simulink model "Drive_Path_Planning"  (R2020a)
settings: Solver=FixedStepAuto  StartTime=0.0  StopTime=30  FixedStep=0.001  RelTol=1e-3  EnableMultiTasking=on
undefined symbols (not defined in the file): gain, sigbuilder_block, X, x_constant, Y, Z
libraries: sm_lib x168, nesl_utility x16, simulink x8, Contact_Forces_Lib x5
(part 4 of 4)

== system Drive_Path_Planning/Try_Spot_3  ==
  DIAGONAL 2 Return : Subsystem
  Diagonal 2 : Subsystem
  Rectangular Joint3 : sm_lib/Joints/Rectangular Joint  JointMode=Normal  SenseConstraintForce=off  SenseConstraintForceX=off  SenseConstraintForceY=off  SenseConstraintForceZ=off  SenseConstraintTorque=off  SenseConstraintTorqueX=off  SenseConstraintTorqueY=off  SenseConstraintTorqueZ=off  SenseTotalForce=off  SenseTotalForceX=off  SenseTotalForceY=off  SenseTotalForceZ=off  SenseTotalTorque=off  SenseTotalTorqueX=off  SenseTotalTorqueY=off  SenseTotalTorqueZ=off  CompositeWrenchDir=FollowerOnBase  CompositeWrenchFrame=BaseFrame  PxEquilibriumPosition=0  PxEquilibriumPositionUnits=m  PxSpringStiffness=0  PxSpringStiffnessUnits=N/m  PxDampingCoefficient=0  PxDampingCoefficientUnits=N/(m/s)  PxTorqueActuationMode=InputTorque  PxMotionActuationMode=ComputedMotion  PxSensePosition=off  PxSenseVelocity=off  PxSenseAcceleration=off  PxSenseTorqueForce=off  PxSenseLowerLimitTorqueForce=off  PxSenseUpperLimitTorqueForce=off  PxLowerLimitSpecify=off  PxLowerLimitBound=-1  PxLowerLimitBoundUnits=m  PxLowerLimitStiffness=1e6  PxLowerLimitStiffnessUnits=N/m  PxLowerLimitDamping=1e3  PxLowerLimitDampingUnits=N/(m/s)  PxLowerLimitTransitionRegionWidth=1e-4  PxLowerLimitTransitionRegionWidthUnits=m  PxUpperLimitSpecify=off  PxUpperLimitBound=1  PxUpperLimitBoundUnits=m  PxUpperLimitStiffness=1e6  PxUpperLimitStiffnessUnits=N/m  PxUpperLimitDamping=1e3  PxUpperLimitDampingUnits=N/(m/s)  PxUpperLimitTransitionRegionWidth=1e-4  PxUpperLimitTransitionRegionWidthUnits=m  PxPositionTargetSpecify=off  PxPositionTargetPriority=High  PxPositionTargetValue=0  PxPositionTargetValueUnits=m  PxVelocityTargetSpecify=off  PxVelocityTargetPriority=High  PxVelocityTargetValue=0  PxVelocityTargetValueUnits=m/s  PyEquilibriumPosition=0  PyEquilibriumPositionUnits=m  PySpringStiffness=0  PySpringStiffnessUnits=N/m  PyDampingCoefficient=0  PyDampingCoefficientUnits=N/(m/s)  PyTorqueActuationMode=InputTorque  PyMotionActuationMode=ComputedMotion  PySensePosition=off  PySenseVelocity=off  PySenseAcceleration=off  PySenseTorqueForce=off  PySenseLowerLimitTorqueForce=off  PySenseUpperLimitTorqueForce=off  PyLowerLimitSpecify=off  PyLowerLimitBound=-1  PyLowerLimitBoundUnits=m  PyLowerLimitStiffness=1e6  PyLowerLimitStiffnessUnits=N/m  PyLowerLimitDamping=1e3  PyLowerLimitDampingUnits=N/(m/s)  PyLowerLimitTransitionRegionWidth=1e-4  PyLowerLimitTransitionRegionWidthUnits=m  PyUpperLimitSpecify=off  PyUpperLimitBound=1  PyUpperLimitBoundUnits=m  PyUpperLimitStiffness=1e6  PyUpperLimitStiffnessUnits=N/m  PyUpperLimitDamping=1e3  PyUpperLimitDampingUnits=N/(m/s)  PyUpperLimitTransitionRegionWidth=1e-4  PyUpperLimitTransitionRegionWidthUnits=m  PyPositionTargetSpecify=off  PyPositionTargetPriority=High  PyPositionTargetValue=0  PyPositionTargetValueUnits=m  PyVelocityTargetSpecify=off  PyVelocityTargetPriority=High  PyVelocityTargetValue=0  PyVelocityTargetValueUnits=m/s
  Rectangular Joint4 : sm_lib/Joints/Rectangular Joint  JointMode=Normal  SenseConstraintForce=off  SenseConstraintForceX=off  SenseConstraintForceY=off  SenseConstraintForceZ=off  SenseConstraintTorque=off  SenseConstraintTorqueX=off  SenseConstraintTorqueY=off  SenseConstraintTorqueZ=off  SenseTotalForce=off  SenseTotalForceX=off  SenseTotalForceY=off  SenseTotalForceZ=off  SenseTotalTorque=off  SenseTotalTorqueX=off  SenseTotalTorqueY=off  SenseTotalTorqueZ=off  CompositeWrenchDir=FollowerOnBase  CompositeWrenchFrame=BaseFrame  PxEquilibriumPosition=0  PxEquilibriumPositionUnits=m  PxSpringStiffness=0  PxSpringStiffnessUnits=N/m  PxDampingCoefficient=0  PxDampingCoefficientUnits=N/(m/s)  PxTorqueActuationMode=InputTorque  PxMotionActuationMode=ComputedMotion  PxSensePosition=off  PxSenseVelocity=off  PxSenseAcceleration=off  PxSenseTorqueForce=off  PxSenseLowerLimitTorqueForce=off  PxSenseUpperLimitTorqueForce=off  PxLowerLimitSpecify=off  PxLowerLimitBound=-1  PxLowerLimitBoundUnits=m  PxLowerLimitStiffness=1e6  PxLowerLimitStiffnessUnits=N/m  PxLowerLimitDamping=1e3  PxLowerLimitDampingUnits=N/(m/s)  PxLowerLimitTransitionRegionWidth=1e-4  PxLowerLimitTransitionRegionWidthUnits=m  PxUpperLimitSpecify=off  PxUpperLimitBound=1  PxUpperLimitBoundUnits=m  PxUpperLimitStiffness=1e6  PxUpperLimitStiffnessUnits=N/m  PxUpperLimitDamping=1e3  PxUpperLimitDampingUnits=N/(m/s)  PxUpperLimitTransitionRegionWidth=1e-4  PxUpperLimitTransitionRegionWidthUnits=m  PxPositionTargetSpecify=off  PxPositionTargetPriority=High  PxPositionTargetValue=0  PxPositionTargetValueUnits=m  PxVelocityTargetSpecify=off  PxVelocityTargetPriority=High  PxVelocityTargetValue=0  PxVelocityTargetValueUnits=m/s  PyEquilibriumPosition=0  PyEquilibriumPositionUnits=m  PySpringStiffness=0  PySpringStiffnessUnits=N/m  PyDampingCoefficient=0  PyDampingCoefficientUnits=N/(m/s)  PyTorqueActuationMode=InputTorque  PyMotionActuationMode=ComputedMotion  PySensePosition=off  PySenseVelocity=off  PySenseAcceleration=off  PySenseTorqueForce=off  PySenseLowerLimitTorqueForce=off  PySenseUpperLimitTorqueForce=off  PyLowerLimitSpecify=off  PyLowerLimitBound=-1  PyLowerLimitBoundUnits=m  PyLowerLimitStiffness=1e6  PyLowerLimitStiffnessUnits=N/m  PyLowerLimitDamping=1e3  PyLowerLimitDampingUnits=N/(m/s)  PyLowerLimitTransitionRegionWidth=1e-4  PyLowerLimitTransitionRegionWidthUnits=m  PyUpperLimitSpecify=off  PyUpperLimitBound=1  PyUpperLimitBoundUnits=m  PyUpperLimitStiffness=1e6  PyUpperLimitStiffnessUnits=N/m  PyUpperLimitDamping=1e3  PyUpperLimitDampingUnits=N/(m/s)  PyUpperLimitTransitionRegionWidth=1e-4  PyUpperLimitTransitionRegionWidthUnits=m  PyPositionTargetSpecify=off  PyPositionTargetPriority=High  PyPositionTargetValue=0  PyPositionTargetValueUnits=m  PyVelocityTargetSpecify=off  PyVelocityTargetPriority=High  PyVelocityTargetValue=0  PyVelocityTargetValueUnits=m/s
  Simulink-PS Converter{5..8} (4 alike) : nesl_utility/Simulink-PS Converter  PhysicalDomain=network_engine_domain  SubClassName=ps_input  LeftPortType=input  RightPortType=output  PseudoPeriodic=off  Frequencies=[]  NoiseDistribution=none  NoiseParameters=[]  Unit=1  AffineConversion=off  FilteringAndDerivatives=provide  SimscapeFilterOrder=1  InputFilterTimeConstant=0.001  UdotUserProvided=0
  Terminator2 : Terminator
  Terminator3 : Terminator
  Conn1 : PMIOPort  Side=Left
  Conn2 : PMIOPort  Port=2  Side=Right
  Conn3 : PMIOPort  Port=3  Side=Left
  Conn4 : PMIOPort  Port=4  Side=Right
  wires:
  Diagonal 2/3(Out3) -> Simulink-PS Converter5/1
  DIAGONAL 2 Return/3(Out3) -> Simulink-PS Converter7/1
  Diagonal 2/4(Out4) -> Simulink-PS Converter6/1
  Diagonal 2/2(Out2) -> Terminator2/1
  Diagonal 2/1(Out1) -> Terminator3/1
  DIAGONAL 2 Return/4(Out4) -> Simulink-PS Converter8/1
  connections:
  Rectangular Joint3/RConn1 -- Conn2/RConn1
  Simulink-PS Converter6/RConn1 -- Rectangular Joint3/LConn3
  Simulink-PS Converter8/RConn1 -- Rectangular Joint4/LConn3
  Rectangular Joint4/LConn1 -- Conn3/RConn1
  Simulink-PS Converter5/RConn1 -- Rectangular Joint3/LConn2
  Simulink-PS Converter7/RConn1 -- Rectangular Joint4/LConn2
  Rectangular Joint4/RConn1 -- Conn4/RConn1
  Rectangular Joint3/LConn1 -- Conn1/RConn1

== system Drive_Path_Planning/Try_Spot_4 ==
  EQUATION PAth1 : Subsystem
  Equation Curve CONSTANT1 : Subsystem
  Rectangular Joint7 : sm_lib/Joints/Rectangular Joint  JointMode=Normal  SenseConstraintForce=off  SenseConstraintForceX=off  SenseConstraintForceY=off  SenseConstraintForceZ=off  SenseConstraintTorque=off  SenseConstraintTorqueX=off  SenseConstraintTorqueY=off  SenseConstraintTorqueZ=off  SenseTotalForce=off  SenseTotalForceX=off  SenseTotalForceY=off  SenseTotalForceZ=off  SenseTotalTorque=off  SenseTotalTorqueX=off  SenseTotalTorqueY=off  SenseTotalTorqueZ=off  CompositeWrenchDir=FollowerOnBase  CompositeWrenchFrame=BaseFrame  PxEquilibriumPosition=0  PxEquilibriumPositionUnits=m  PxSpringStiffness=0  PxSpringStiffnessUnits=N/m  PxDampingCoefficient=0  PxDampingCoefficientUnits=N/(m/s)  PxTorqueActuationMode=InputTorque  PxMotionActuationMode=ComputedMotion  PxSensePosition=off  PxSenseVelocity=off  PxSenseAcceleration=off  PxSenseTorqueForce=off  PxSenseLowerLimitTorqueForce=off  PxSenseUpperLimitTorqueForce=off  PxLowerLimitSpecify=off  PxLowerLimitBound=-1  PxLowerLimitBoundUnits=m  PxLowerLimitStiffness=1e6  PxLowerLimitStiffnessUnits=N/m  PxLowerLimitDamping=1e3  PxLowerLimitDampingUnits=N/(m/s)  PxLowerLimitTransitionRegionWidth=1e-4  PxLowerLimitTransitionRegionWidthUnits=m  PxUpperLimitSpecify=off  PxUpperLimitBound=6.1  PxUpperLimitBoundUnits=m  PxUpperLimitStiffness=1e10  PxUpperLimitStiffnessUnits=N/m  PxUpperLimitDamping=1e3  PxUpperLimitDampingUnits=N/(m/s)  PxUpperLimitTransitionRegionWidth=1e-4  PxUpperLimitTransitionRegionWidthUnits=m  PxPositionTargetSpecify=off  PxPositionTargetPriority=High  PxPositionTargetValue=0  PxPositionTargetValueUnits=m  PxVelocityTargetSpecify=off  PxVelocityTargetPriority=High  PxVelocityTargetValue=0  PxVelocityTargetValueUnits=m/s  PyEquilibriumPosition=0  PyEquilibriumPositionUnits=m  PySpringStiffness=0  PySpringStiffnessUnits=N/m  PyDampingCoefficient=0  PyDampingCoefficientUnits=N/(m/s)  PyTorqueActuationMode=InputTorque  PyMotionActuationMode=ComputedMotion  PySensePosition=off  PySenseVelocity=off  PySenseAcceleration=off  PySenseTorqueForce=off  PySenseLowerLimitTorqueForce=off  PySenseUpperLimitTorqueForce=off  PyLowerLimitSpecify=off  PyLowerLimitBound=-1  PyLowerLimitBoundUnits=m  PyLowerLimitStiffness=1e6  PyLowerLimitStiffnessUnits=N/m  PyLowerLimitDamping=1e3  PyLowerLimitDampingUnits=N/(m/s)  PyLowerLimitTransitionRegionWidth=1e-4  PyLowerLimitTransitionRegionWidthUnits=m  PyUpperLimitSpecify=off  PyUpperLimitBound=8.455  PyUpperLimitBoundUnits=m  PyUpperLimitStiffness=1e6  PyUpperLimitStiffnessUnits=N/m  PyUpperLimitDamping=1e3  PyUpperLimitDampingUnits=N/(m/s)  PyUpperLimitTransitionRegionWidth=1e-4  PyUpperLimitTransitionRegionWidthUnits=m  PyPositionTargetSpecify=off  PyPositionTargetPriority=High  PyPositionTargetValue=0  PyPositionTargetValueUnits=m  PyVelocityTargetSpecify=off  PyVelocityTargetPriority=High  PyVelocityTargetValue=1.1  PyVelocityTargetValueUnits=m/s
  Simulink-PS Converter10 : nesl_utility/Simulink-PS Converter  PhysicalDomain=network_engine_domain  SubClassName=ps_input  LeftPortType=input  RightPortType=output  PseudoPeriodic=off  Frequencies=[]  NoiseDistribution=none  NoiseParameters=[]  Unit=1  AffineConversion=off  FilteringAndDerivatives=provide  SimscapeFilterOrder=1  InputFilterTimeConstant=0.001  UdotUserProvided=0
  Conn1 : PMIOPort  Side=Right
  Conn2 : PMIOPort  Port=2  Side=Left
  Conn3 : PMIOPort  Port=3  Side=Left
  wires:
  EQUATION PAth1/1(Out1) -> Simulink-PS Converter10/1
  connections:
  Simulink-PS Converter10/RConn1 -- Rectangular Joint7/LConn3
  Rectangular Joint7/LConn1 -- Conn2/RConn1
  Equation Curve CONSTANT1/RConn1 -- Rectangular Joint7/LConn2
  Rectangular Joint7/RConn1 -- Conn1/RConn1
  EQUATION PAth1/LConn1 -- Conn3/RConn1

== system Drive_Path_Planning/ /Signal Builder ==
  Demux : Demux  Tag=STV Demux  Outputs=2
      settings: DisplayOption=none
  FromWs : FromWorkspace  Tag=STV FromWs  VariableName=tuvar
      SigBuilderData=|
      | common.afterFinalStr = 'Extrapolate'
      | common.sampleTime = 0
      | dataSet.timeRange = [0 10]
      | dataSet.name = 'Group 1'
      | sbobj.Groups.Name = 'Group 1'
      | sbobj.Groups.Signals(1).Name = 'S2'
      | sbobj.Groups.Signals(1).XData = [0 0.4 0.4 5 5 10]
      | sbobj.Groups.Signals(1).YData = [0 0 -0.02 -0.02 0 0]
      | sbobj.Groups.Signals(2).Name = '1'
      | sbobj.Groups.Signals(2).XData = [0 0.2 0.2 0.4 0.4 10]
      | sbobj.Groups.Signals(2).YData = [0 0 10 10 0 0]
  S2 : Outport  Tag=STV Outport
  1 : Outport  Tag=STV Outport  Port=2
  wires:
  FromWs/1 -> Demux/1
  Demux/1 -> S2/1
  Demux/2 -> 1/1

== system Drive_Path_Planning/ Try_Spot_5 /EQUATION PAth ==
  Clock4 : Clock
  If Action Subsystem6 : Subsystem  TreatAsAtomicUnit=on
  If5 : If  IfExpression=u1>20
  Multiply1 : Gain  Gain=gain
  Subsystem5 : Subsystem
  Subsystem6 : Subsystem
  Subsystem7 : Subsystem
  Conn1 : PMIOPort  Side=Left
  Out1 : Outport
  Out2 : Outport  Port=2
  wires:
  Multiply1/1 -> If Action Subsystem6/1(In1)
  Subsystem5/1(Out1) -> Subsystem6/1(In1)
  If5/1 -> If Action Subsystem6/Action
  Subsystem6/1(Out1) -> Subsystem7/1(In1)
  Subsystem7/1(Out1) -> Multiply1/1
  If5/2 -> Out2/1
  Clock4/1 -> If5/1
  If Action Subsystem6/1(Out1) -> Out1/1
  connections:
  Subsystem5/LConn1 -- Conn1/RConn1

== system Drive_Path_Planning/ Try_Spot_5 /Equation Curve CONSTANT ==
  Clock1 : Clock
  Constant7 : Constant  Value=38
  If Action Subsystem3 : Subsystem  TreatAsAtomicUnit=on
  If3 : If  IfExpression=u1 > 20
  Product4 : Product
  Signal Builder4 : Subsystem  Tag=STV Subsys  LoadFcn=sigbuilder_block('load');  StartFcn=sigbuilder_block('start');  StopFcn=sigbuilder_block('stop');  ClipboardFcn=sigbuilder_block('clipboard');  mask(Sigbuilder block){tuvar=[0:10]}
      mask help: Simulink:masks:SigbuilderBlock_MD
      mask init:
      | if ~strcmp(get_param(bdroot(gcbh),'SimulationStatus'),'stopped') tuvar = sigbuilder_block('maskInit'); end
      settings: CopyFcn=sigbuilder_block('copy');  DeleteFcn=sigbuilder_block('delete');  ModelCloseFcn=sigbuilder_block('modelClose');  PreSaveFcn=sigbuilder_block('preSave');  PauseFcn=sigbuilder_block('pause');  ContinueFcn=sigbuilder_block('continue');  NameChangeFcn=sigbuilder_block('namechange');  OpenFcn=sigbuilder_block('open',[437.6 153 550.4 359.25 ]);  CloseFcn=sigbuilder_block('close');
      mask Display: plot(0, 0, 100, 100,[2, 2, 32, 32, 2], [68, 8, 8, 68, 68],[32, 2], [38, 38], [32, 19, 2],[53, 60, 44], [32, 17, 17, 2],[16, 16, 31, 31]);txt = getActiveGroup(gcbh);text(2, 100, txt,'verticalAlignment', 'top');
  Simulink-PS Converter11 : nesl_utility/Simulink-PS Converter  PhysicalDomain=network_engine_domain  SubClassName=ps_input  LeftPortType=input  RightPortType=output  PseudoPeriodic=off  Frequencies=[]  NoiseDistribution=none  NoiseParameters=[]  Unit=1  AffineConversion=off  FilteringAndDerivatives=provide  SimscapeFilterOrder=1  InputFilterTimeConstant=0.001  UdotUserProvided=0
  Conn1 : PMIOPort  Side=Right
  Out1 : Outport
  wires:
  Product4/1 -> If Action Subsystem3/1(In1)
  If3/1 -> If Action Subsystem3/Action
  Constant7/1 -> Product4/2
  Clock1/1 -> If3/1
  Signal Builder4/1(Signal 1) -> Product4/1
  If3/2 -> Out1/1
  If Action Subsystem3/1(Out1) -> Simulink-PS Converter11/1
  connections:
  Simulink-PS Converter11/RConn1 -- Conn1/RConn1

== system Drive_Path_Planning/BOT/Friction_Wheel_1 ==
  Sphere to Plane Force : Contact_Forces_Lib/3D/Sphere to Plane Force  sphere_rad=0.063  plane_lenx=13.3  plane_leny=10  plane_depth=0.00005  force_law=Linear  k_contact=1e4  b_contact=1e2  pen_full_damp_F=1e-4  pen_exponent=1  custom_param_1=1  custom_param_2=1  friction_law=Stick-Slip Continuous  mu_kinetic=friction  mu_static=0.4  v_thr=0.1  vis_on=off  vis_opc_en=0  vis_len_plaBz=0.005  vis_clr=[0.9 0.2 0.2]  vis_opc=0.7
  Terminator : Terminator
  Conn2 : PMIOPort  Side=Left
  Cylindrical Solid26 : PMIOPort  Port=2  Side=Left
  wires:
  Sphere to Plane Force/1 -> Terminator/1
  connections:
  Sphere to Plane Force/RConn1 -- Conn2/RConn1
  Cylindrical Solid26/RConn1 -- Sphere to Plane Force/LConn1

== system Drive_Path_Planning/BOT/Friction_Wheel_2 ==
  Sphere to Plane Force1 : Contact_Forces_Lib/3D/Sphere to Plane Force  sphere_rad=0.063  plane_lenx=13.3  plane_leny=10  plane_depth=0.00005  force_law=Linear  k_contact=1e4  b_contact=1e2  pen_full_damp_F=1e-4  pen_exponent=1  custom_param_1=1  custom_param_2=1  friction_law=Stick-Slip Continuous  mu_kinetic=friction  mu_static=0.4  v_thr=0.1  vis_on=off  vis_opc_en=0  vis_len_plaBz=0.005  vis_clr=[0.9 0.2 0.2]  vis_opc=0.7
  Sphere to Plane Force3 : Contact_Forces_Lib/3D/Sphere to Plane Force  sphere_rad=0.78  plane_lenx=0.8005  plane_leny=1.2375  plane_depth=0.05  force_law=Linear  k_contact=1e4  b_contact=1e2  pen_full_damp_F=1e-4  pen_exponent=1  custom_param_1=1  custom_param_2=1  friction_law=Stick-Slip Continuous  mu_kinetic=friction_1  mu_static=0.09  v_thr=0.001  vis_on=off  vis_opc_en=0  vis_len_plaBz=0.005  vis_clr=[0.9 0.2 0.2]  vis_opc=0.7
  Terminator1 : Terminator
  Terminator3 : Terminator
  Conn4 : PMIOPort  Side=Left
  Connection Port : PMIOPort  Port=2  Side=Left
  Cylindrical Solid26 : PMIOPort  Port=3  Side=Left
  wires:
  Sphere to Plane Force1/1 -> Terminator1/1
  Sphere to Plane Force3/1 -> Terminator3/1
  connections:
  Sphere to Plane Force1/LConn1 -- Cylindrical Solid26/RConn1 -- Sphere to Plane Force3/LConn1
  Sphere to Plane Force3/RConn1 -- Connection Port/RConn1
  Conn4/RConn1 -- Sphere to Plane Force1/RConn1

== system Drive_Path_Planning/BOT/Friction_Wheel_3 ==
  Sphere to Plane Force2 : Contact_Forces_Lib/3D/Sphere to Plane Force  sphere_rad=0.063  plane_lenx=13.3  plane_leny=10  plane_depth=0.00005  force_law=Linear  k_contact=1e4  b_contact=1e2  pen_full_damp_F=1e-4  pen_exponent=1  custom_param_1=1  custom_param_2=1  friction_law=Stick-Slip Continuous  mu_kinetic=friction  mu_static=0.4  v_thr=0.1  vis_on=off  vis_opc_en=0  vis_len_plaBz=0.005  vis_clr=[0.9 0.2 0.2]  vis_opc=0.7
  Sphere to Plane Force4 : Contact_Forces_Lib/3D/Sphere to Plane Force  sphere_rad=0.7  plane_lenx=1.2375  plane_leny=1.2375  plane_depth=0.05  force_law=Linear  k_contact=1e4  b_contact=1e2  pen_full_damp_F=1e-4  pen_exponent=1  custom_param_1=1  custom_param_2=1  friction_law=Stick-Slip Continuous  mu_kinetic=friction_2  mu_static=0.09  v_thr=0.001  vis_on=off  vis_opc_en=0  vis_len_plaBz=0.005  vis_clr=[0.9 0.2 0.2]  vis_opc=0.7
  Terminator : Terminator
  Terminator2 : Terminator
  Cylindrical Solid27 : PMIOPort  Side=Left
  Conn3 : PMIOPort  Port=2  Side=Left
  Conn5 : PMIOPort  Port=3  Side=Left
  wires:
  Sphere to Plane Force2/1 -> Terminator2/1
  Sphere to Plane Force4/1 -> Terminator/1
  connections:
  Sphere to Plane Force2/LConn1 -- Cylindrical Solid27/RConn1 -- Sphere to Plane Force4/LConn1
  Conn3/RConn1 -- Sphere to Plane Force2/RConn1
  Conn5/RConn1 -- Sphere to Plane Force4/RConn1

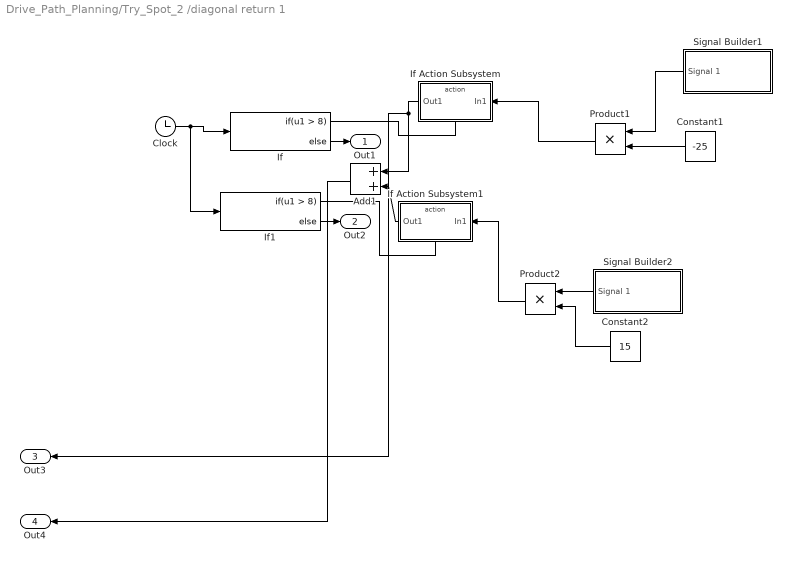
== system Drive_Path_Planning/Try_Spot_2 /diagonal return 1 ==
  Add1 : Sum
  Clock : Clock
  Constant1 : Constant  Value=-25
  Constant2 : Constant  Value=15
  If : If  IfExpression=u1 > 8
  If Action Subsystem : Subsystem  TreatAsAtomicUnit=on
  If Action Subsystem1 : Subsystem  TreatAsAtomicUnit=on
  If1 : If  IfExpression=u1 > 8
  Product1 : Product
  Product2 : Product
  Signal Builder1 : Subsystem  Tag=STV Subsys  LoadFcn=sigbuilder_block('load');  StartFcn=sigbuilder_block('start');  StopFcn=sigbuilder_block('stop');  ClipboardFcn=sigbuilder_block('clipboard');  mask(Sigbuilder block){tuvar=[0:10]}
      mask help: Simulink:masks:SigbuilderBlock_MD
      mask init:
      | if ~strcmp(get_param(bdroot(gcbh),'SimulationStatus'),'stopped') tuvar = sigbuilder_block('maskInit'); end
      settings: CopyFcn=sigbuilder_block('copy');  DeleteFcn=sigbuilder_block('delete');  ModelCloseFcn=sigbuilder_block('modelClose');  PreSaveFcn=sigbuilder_block('preSave');  PauseFcn=sigbuilder_block('pause');  ContinueFcn=sigbuilder_block('continue');  NameChangeFcn=sigbuilder_block('namechange');  OpenFcn=sigbuilder_block('open',[437.6 153 550.4 359.25 ]);  CloseFcn=sigbuilder_block('close');
      mask Display: plot(0, 0, 100, 100,[2, 2, 32, 32, 2], [68, 8, 8, 68, 68],[32, 2], [38, 38], [32, 19, 2],[53, 60, 44], [32, 17, 17, 2],[16, 16, 31, 31]);txt = getActiveGroup(gcbh);text(2, 100, txt,'verticalAlignment', 'top');
  Signal Builder2 : Subsystem  Tag=STV Subsys  LoadFcn=sigbuilder_block('load');  StartFcn=sigbuilder_block('start');  StopFcn=sigbuilder_block('stop');  ClipboardFcn=sigbuilder_block('clipboard');  mask(Sigbuilder block){tuvar=[0:10]}
      mask help: Simulink:masks:SigbuilderBlock_MD
      mask init:
      | if ~strcmp(get_param(bdroot(gcbh),'SimulationStatus'),'stopped') tuvar = sigbuilder_block('maskInit'); end
      settings: CopyFcn=sigbuilder_block('copy');  DeleteFcn=sigbuilder_block('delete');  ModelCloseFcn=sigbuilder_block('modelClose');  PreSaveFcn=sigbuilder_block('preSave');  PauseFcn=sigbuilder_block('pause');  ContinueFcn=sigbuilder_block('continue');  NameChangeFcn=sigbuilder_block('namechange');  OpenFcn=sigbuilder_block('open',[437.6 153 550.4 359.25 ]);  CloseFcn=sigbuilder_block('close');
      mask Display: plot(0, 0, 100, 100,[2, 2, 32, 32, 2], [68, 8, 8, 68, 68],[32, 2], [38, 38], [32, 19, 2],[53, 60, 44], [32, 17, 17, 2],[16, 16, 31, 31]);txt = getActiveGroup(gcbh);text(2, 100, txt,'verticalAlignment', 'top');
  Out1 : Outport
  Out2 : Outport  Port=2
  Out3 : Outport  Port=3
  Out4 : Outport  Port=4
  wires:
  Constant1/1 -> Product1/2
  If Action Subsystem1/1(Out1) -> Add1/2
  Signal Builder2/1(Signal 1) -> Product2/1
  If/2 -> Out1/1
  Product2/1 -> If Action Subsystem1/1(In1)
  If Action Subsystem/1(Out1) -> Out3/1, Add1/1
  Constant2/1 -> Product2/2
  Product1/1 -> If Action Subsystem/1(In1)
  Add1/1 -> Out4/1
  Clock/1 -> If1/1, If/1
  Signal Builder1/1(Signal 1) -> Product1/1
  If1/2 -> Out2/1
  If/1 -> If Action Subsystem/Action
  If1/1 -> If Action Subsystem1/Action

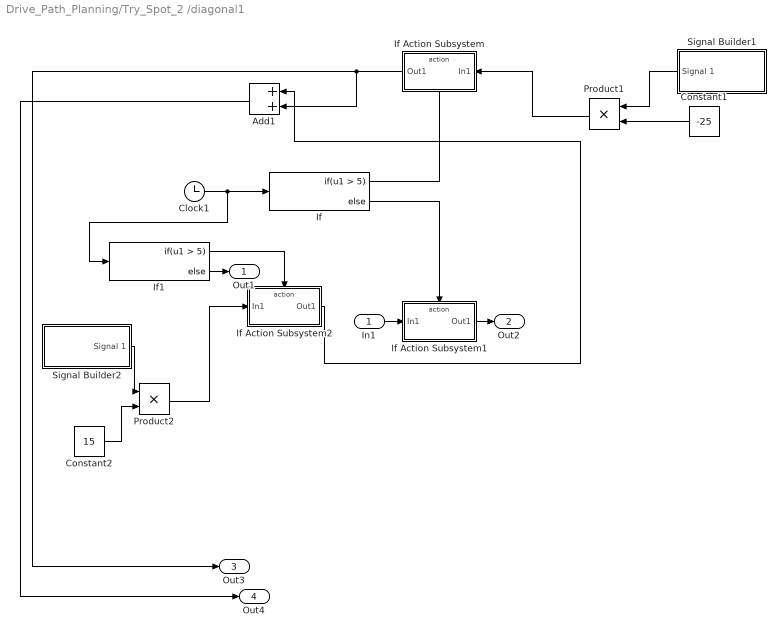
== system Drive_Path_Planning/Try_Spot_2 /diagonal1 ==
  In1 : Inport
  Add1 : Sum
  Clock1 : Clock
  Constant1 : Constant  Value=-25
  Constant2 : Constant  Value=15
  If : If  IfExpression=u1 > 5
  If Action Subsystem : Subsystem  TreatAsAtomicUnit=on
  If Action Subsystem1 : Subsystem  TreatAsAtomicUnit=on
  If Action Subsystem2 : Subsystem  TreatAsAtomicUnit=on
  If1 : If  IfExpression=u1 > 5
  Product1 : Product
  Product2 : Product
  Signal Builder1 : Subsystem  Tag=STV Subsys  LoadFcn=sigbuilder_block('load');  StartFcn=sigbuilder_block('start');  StopFcn=sigbuilder_block('stop');  ClipboardFcn=sigbuilder_block('clipboard');  mask(Sigbuilder block){tuvar=[0:10]}
      mask help: Simulink:masks:SigbuilderBlock_MD
      mask init:
      | if ~strcmp(get_param(bdroot(gcbh),'SimulationStatus'),'stopped') tuvar = sigbuilder_block('maskInit'); end
      settings: CopyFcn=sigbuilder_block('copy');  DeleteFcn=sigbuilder_block('delete');  ModelCloseFcn=sigbuilder_block('modelClose');  PreSaveFcn=sigbuilder_block('preSave');  PauseFcn=sigbuilder_block('pause');  ContinueFcn=sigbuilder_block('continue');  NameChangeFcn=sigbuilder_block('namechange');  OpenFcn=sigbuilder_block('open',[437.6 153 550.4 359.25 ]);  CloseFcn=sigbuilder_block('close');
      mask Display: plot(0, 0, 100, 100,[2, 2, 32, 32, 2], [68, 8, 8, 68, 68],[32, 2], [38, 38], [32, 19, 2],[53, 60, 44], [32, 17, 17, 2],[16, 16, 31, 31]);txt = getActiveGroup(gcbh);text(2, 100, txt,'verticalAlignment', 'top');
  Signal Builder2 : Subsystem  Tag=STV Subsys  LoadFcn=sigbuilder_block('load');  StartFcn=sigbuilder_block('start');  StopFcn=sigbuilder_block('stop');  ClipboardFcn=sigbuilder_block('clipboard');  mask(Sigbuilder block){tuvar=[0:10]}
      mask help: Simulink:masks:SigbuilderBlock_MD
      mask init:
      | if ~strcmp(get_param(bdroot(gcbh),'SimulationStatus'),'stopped') tuvar = sigbuilder_block('maskInit'); end
      settings: CopyFcn=sigbuilder_block('copy');  DeleteFcn=sigbuilder_block('delete');  ModelCloseFcn=sigbuilder_block('modelClose');  PreSaveFcn=sigbuilder_block('preSave');  PauseFcn=sigbuilder_block('pause');  ContinueFcn=sigbuilder_block('continue');  NameChangeFcn=sigbuilder_block('namechange');  OpenFcn=sigbuilder_block('open',[437.6 153 550.4 359.25 ]);  CloseFcn=sigbuilder_block('close');
      mask Display: plot(0, 0, 100, 100,[2, 2, 32, 32, 2], [68, 8, 8, 68, 68],[32, 2], [38, 38], [32, 19, 2],[53, 60, 44], [32, 17, 17, 2],[16, 16, 31, 31]);txt = getActiveGroup(gcbh);text(2, 100, txt,'verticalAlignment', 'top');
  Out1 : Outport
  Out2 : Outport  Port=2
  Out3 : Outport  Port=3
  Out4 : Outport  Port=4
  wires:
  Product2/1 -> If Action Subsystem2/1(In1)
  If Action Subsystem/1(Out1) -> Out3/1, Add1/2
  If/1 -> If Action Subsystem/Action
  Clock1/1 -> If1/1, If/1
  If/2 -> If Action Subsystem1/Action
  Signal Builder2/1(Signal 1) -> Product2/1
  If1/1 -> If Action Subsystem2/Action
  If Action Subsystem2/1(Out1) -> Add1/1
  In1/1 -> If Action Subsystem1/1(In1)
  Constant1/1 -> Product1/2
  Product1/1 -> If Action Subsystem/1(In1)
  Constant2/1 -> Product2/2
  Signal Builder1/1(Signal 1) -> Product1/1
  Add1/1 -> Out4/1
  If Action Subsystem1/1(Out1) -> Out2/1
  If1/2 -> Out1/1

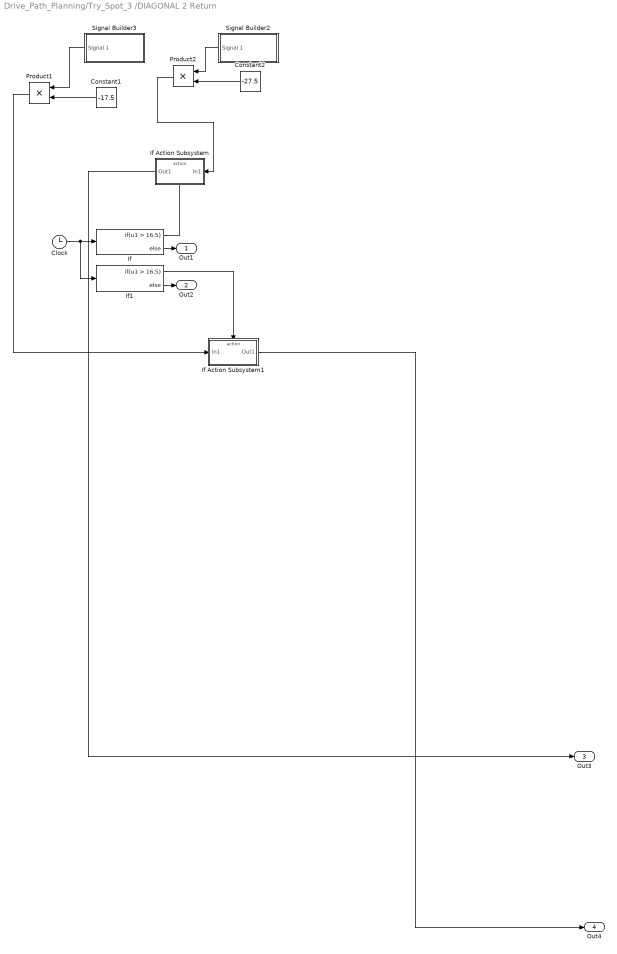
== system Drive_Path_Planning/Try_Spot_3 /DIAGONAL 2 Return ==
  Clock : Clock
  Constant1 : Constant  Value=-17.5
  Constant2 : Constant  Value=-27.5
  If : If  IfExpression=u1 > 16.5
  If Action Subsystem : Subsystem  TreatAsAtomicUnit=on
  If Action Subsystem1 : Subsystem  TreatAsAtomicUnit=on
  If1 : If  IfExpression=u1 > 16.5
  Product1 : Product
  Product2 : Product
  Signal Builder2 : Subsystem  Tag=STV Subsys  LoadFcn=sigbuilder_block('load');  StartFcn=sigbuilder_block('start');  StopFcn=sigbuilder_block('stop');  ClipboardFcn=sigbuilder_block('clipboard');  mask(Sigbuilder block){tuvar=[0:10]}
      mask help: Simulink:masks:SigbuilderBlock_MD
      mask init:
      | if ~strcmp(get_param(bdroot(gcbh),'SimulationStatus'),'stopped') tuvar = sigbuilder_block('maskInit'); end
      settings: CopyFcn=sigbuilder_block('copy');  DeleteFcn=sigbuilder_block('delete');  ModelCloseFcn=sigbuilder_block('modelClose');  PreSaveFcn=sigbuilder_block('preSave');  PauseFcn=sigbuilder_block('pause');  ContinueFcn=sigbuilder_block('continue');  NameChangeFcn=sigbuilder_block('namechange');  OpenFcn=sigbuilder_block('open',[437.6 153 550.4 359.25 ]);  CloseFcn=sigbuilder_block('close');
      mask Display: plot(0, 0, 100, 100,[2, 2, 32, 32, 2], [68, 8, 8, 68, 68],[32, 2], [38, 38], [32, 19, 2],[53, 60, 44], [32, 17, 17, 2],[16, 16, 31, 31]);txt = getActiveGroup(gcbh);text(2, 100, txt,'verticalAlignment', 'top');
  Signal Builder3 : Subsystem  Tag=STV Subsys  LoadFcn=sigbuilder_block('load');  StartFcn=sigbuilder_block('start');  StopFcn=sigbuilder_block('stop');  ClipboardFcn=sigbuilder_block('clipboard');  mask(Sigbuilder block){tuvar=[0:10]}
      mask help: Simulink:masks:SigbuilderBlock_MD
      mask init:
      | if ~strcmp(get_param(bdroot(gcbh),'SimulationStatus'),'stopped') tuvar = sigbuilder_block('maskInit'); end
      settings: CopyFcn=sigbuilder_block('copy');  DeleteFcn=sigbuilder_block('delete');  ModelCloseFcn=sigbuilder_block('modelClose');  PreSaveFcn=sigbuilder_block('preSave');  PauseFcn=sigbuilder_block('pause');  ContinueFcn=sigbuilder_block('continue');  NameChangeFcn=sigbuilder_block('namechange');  OpenFcn=sigbuilder_block('open',[437.6 153 550.4 359.25 ]);  CloseFcn=sigbuilder_block('close');
      mask Display: plot(0, 0, 100, 100,[2, 2, 32, 32, 2], [68, 8, 8, 68, 68],[32, 2], [38, 38], [32, 19, 2],[53, 60, 44], [32, 17, 17, 2],[16, 16, 31, 31]);txt = getActiveGroup(gcbh);text(2, 100, txt,'verticalAlignment', 'top');
  Out1 : Outport
  Out2 : Outport  Port=2
  Out3 : Outport  Port=3
  Out4 : Outport  Port=4
  wires:
  Signal Builder3/1(Signal 1) -> Product1/1
  Constant1/1 -> Product1/2
  If1/1 -> If Action Subsystem1/Action
  Product1/1 -> If Action Subsystem1/1(In1)
  If/1 -> If Action Subsystem/Action
  Clock/1 -> If1/1, If/1
  Product2/1 -> If Action Subsystem/1(In1)
  If/2 -> Out1/1
  Constant2/1 -> Product2/2
  Signal Builder2/1(Signal 1) -> Product2/1
  If1/2 -> Out2/1
  If Action Subsystem1/1(Out1) -> Out4/1
  If Action Subsystem/1(Out1) -> Out3/1

== system Drive_Path_Planning/Try_Spot_3 /Diagonal 2 ==
  Clock : Clock
  Constant1 : Constant  Value=-17
  Constant2 : Constant  Value=-25
  If : If  IfExpression=u1 > 13
  If Action Subsystem : Subsystem  TreatAsAtomicUnit=on
  If Action Subsystem1 : Subsystem  TreatAsAtomicUnit=on
  If1 : If  IfExpression=u1 > 13
  Product1 : Product
  Product2 : Product
  Signal Builder1 : Subsystem  Tag=STV Subsys  LoadFcn=sigbuilder_block('load');  StartFcn=sigbuilder_block('start');  StopFcn=sigbuilder_block('stop');  ClipboardFcn=sigbuilder_block('clipboard');  mask(Sigbuilder block){tuvar=[0:10]}
      mask help: Simulink:masks:SigbuilderBlock_MD
      mask init:
      | if ~strcmp(get_param(bdroot(gcbh),'SimulationStatus'),'stopped') tuvar = sigbuilder_block('maskInit'); end
      settings: CopyFcn=sigbuilder_block('copy');  DeleteFcn=sigbuilder_block('delete');  ModelCloseFcn=sigbuilder_block('modelClose');  PreSaveFcn=sigbuilder_block('preSave');  PauseFcn=sigbuilder_block('pause');  ContinueFcn=sigbuilder_block('continue');  NameChangeFcn=sigbuilder_block('namechange');  OpenFcn=sigbuilder_block('open',[437.6 153 550.4 359.25 ]);  CloseFcn=sigbuilder_block('close');
      mask Display: plot(0, 0, 100, 100,[2, 2, 32, 32, 2], [68, 8, 8, 68, 68],[32, 2], [38, 38], [32, 19, 2],[53, 60, 44], [32, 17, 17, 2],[16, 16, 31, 31]);txt = getActiveGroup(gcbh);text(2, 100, txt,'verticalAlignment', 'top');
  Signal Builder2 : Subsystem  Tag=STV Subsys  LoadFcn=sigbuilder_block('load');  StartFcn=sigbuilder_block('start');  StopFcn=sigbuilder_block('stop');  ClipboardFcn=sigbuilder_block('clipboard');  mask(Sigbuilder block){tuvar=[0:10]}
      mask help: Simulink:masks:SigbuilderBlock_MD
      mask init:
      | if ~strcmp(get_param(bdroot(gcbh),'SimulationStatus'),'stopped') tuvar = sigbuilder_block('maskInit'); end
      settings: CopyFcn=sigbuilder_block('copy');  DeleteFcn=sigbuilder_block('delete');  ModelCloseFcn=sigbuilder_block('modelClose');  PreSaveFcn=sigbuilder_block('preSave');  PauseFcn=sigbuilder_block('pause');  ContinueFcn=sigbuilder_block('continue');  NameChangeFcn=sigbuilder_block('namechange');  OpenFcn=sigbuilder_block('open',[437.6 153 550.4 359.25 ]);  CloseFcn=sigbuilder_block('close');
      mask Display: plot(0, 0, 100, 100,[2, 2, 32, 32, 2], [68, 8, 8, 68, 68],[32, 2], [38, 38], [32, 19, 2],[53, 60, 44], [32, 17, 17, 2],[16, 16, 31, 31]);txt = getActiveGroup(gcbh);text(2, 100, txt,'verticalAlignment', 'top');
  Out1 : Outport
  Out2 : Outport  Port=2
  Out3 : Outport  Port=3
  Out4 : Outport  Port=4
  wires:
  Product2/1 -> If Action Subsystem/1(In1)
  Signal Builder2/1(Signal 1) -> Product2/1
  Constant2/1 -> Product2/2
  If/1 -> If Action Subsystem/Action
  If/2 -> Out1/1
  If1/1 -> If Action Subsystem1/Action
  Clock/1 -> If1/1, If/1
  Signal Builder1/1(Signal 1) -> Product1/1
  Constant1/1 -> Product1/2
  Product1/1 -> If Action Subsystem1/1(In1)
  If1/2 -> Out2/1
  If Action Subsystem/1(Out1) -> Out3/1
  If Action Subsystem1/1(Out1) -> Out4/1

== system Drive_Path_Planning/Try_Spot_4/EQUATION PAth1 ==
  Clock4 : Clock
  If Action Subsystem6 : Subsystem  TreatAsAtomicUnit=on
  If5 : If  IfExpression=u1>20
  Multiply1 : Gain  Gain=gain
  Subsystem5 : Subsystem
  Subsystem6 : Subsystem
  Subsystem7 : Subsystem
  Conn1 : PMIOPort  Side=Left
  Out1 : Outport
  Out2 : Outport  Port=2
  wires:
  Multiply1/1 -> If Action Subsystem6/1(In1)
  Subsystem5/1(Out1) -> Subsystem6/1(In1)
  If5/1 -> If Action Subsystem6/Action
  Subsystem6/1(Out1) -> Subsystem7/1(In1)
  Subsystem7/1(Out1) -> Multiply1/1
  If5/2 -> Out2/1
  Clock4/1 -> If5/1
  If Action Subsystem6/1(Out1) -> Out1/1
  connections:
  Subsystem5/LConn1 -- Conn1/RConn1

== system Drive_Path_Planning/Try_Spot_4/Equation Curve CONSTANT1 ==
  Clock1 : Clock
  Constant7 : Constant  Value=x_constant
  If Action Subsystem3 : Subsystem  TreatAsAtomicUnit=on
  If3 : If  IfExpression=u1 > 20
  Product4 : Product
  Signal Builder4 : Subsystem  Tag=STV Subsys  LoadFcn=sigbuilder_block('load');  StartFcn=sigbuilder_block('start');  StopFcn=sigbuilder_block('stop');  ClipboardFcn=sigbuilder_block('clipboard');  mask(Sigbuilder block){tuvar=[0:10]}
      mask help: Simulink:masks:SigbuilderBlock_MD
      mask init:
      | if ~strcmp(get_param(bdroot(gcbh),'SimulationStatus'),'stopped') tuvar = sigbuilder_block('maskInit'); end
      settings: CopyFcn=sigbuilder_block('copy');  DeleteFcn=sigbuilder_block('delete');  ModelCloseFcn=sigbuilder_block('modelClose');  PreSaveFcn=sigbuilder_block('preSave');  PauseFcn=sigbuilder_block('pause');  ContinueFcn=sigbuilder_block('continue');  NameChangeFcn=sigbuilder_block('namechange');  OpenFcn=sigbuilder_block('open',[437.6 153 550.4 359.25 ]);  CloseFcn=sigbuilder_block('close');
      mask Display: plot(0, 0, 100, 100,[2, 2, 32, 32, 2], [68, 8, 8, 68, 68],[32, 2], [38, 38], [32, 19, 2],[53, 60, 44], [32, 17, 17, 2],[16, 16, 31, 31]);txt = getActiveGroup(gcbh);text(2, 100, txt,'verticalAlignment', 'top');
  Simulink-PS Converter11 : nesl_utility/Simulink-PS Converter  PhysicalDomain=network_engine_domain  SubClassName=ps_input  LeftPortType=input  RightPortType=output  PseudoPeriodic=off  Frequencies=[]  NoiseDistribution=none  NoiseParameters=[]  Unit=1  AffineConversion=off  FilteringAndDerivatives=provide  SimscapeFilterOrder=1  InputFilterTimeConstant=0.001  UdotUserProvided=0
  Conn1 : PMIOPort  Side=Right
  Out1 : Outport
  wires:
  Product4/1 -> If Action Subsystem3/1(In1)
  If3/1 -> If Action Subsystem3/Action
  Constant7/1 -> Product4/2
  Clock1/1 -> If3/1
  Signal Builder4/1(Signal 1) -> Product4/1
  If3/2 -> Out1/1
  If Action Subsystem3/1(Out1) -> Simulink-PS Converter11/1
  connections:
  Simulink-PS Converter11/RConn1 -- Conn1/RConn1

== system Drive_Path_Planning/ Try_Spot_5 /EQUATION PAth/If Action Subsystem6 ==
  In1 : Inport
  Action Port : ActionPort  ActionPortLabel=if(u1>20)
  Out1 : Outport
  wires:
  In1/1 -> Out1/1

== system Drive_Path_Planning/ Try_Spot_5 /EQUATION PAth/Subsystem5 ==
  Abs : Abs
  Add1 : Sum
  Constant3 : Constant  Value=0.525
  Constant4 : Constant  Value=5.2
  Constant5 : Constant  Value=-2.5
  PS-Simulink Converter : nesl_utility/PS-Simulink Converter  PhysicalDomain=network_engine_domain  SubClassName=ps_output  LeftPortType=input  RightPortType=output  PseudoPeriodic=off  Frequencies=[]  Unit=inherit  AffineConversion=off
  Product3 : Product
  Sqrt : Sqrt  OutputSignalType=real  SaturateOnIntegerOverflow=on
  Subtract : Sum  Inputs=+-
  Conn1 : PMIOPort  Side=Left
  Out1 : Outport
  wires:
  Constant4/1 -> Product3/2
  Sqrt/1 -> Add1/1
  Subtract/1 -> Product3/1
  Product3/1 -> Abs/1
  Abs/1 -> Sqrt/1
  Constant5/1 -> Add1/2
  Constant3/1 -> Subtract/2
  PS-Simulink Converter/1 -> Subtract/1
  Add1/1 -> Out1/1
  connections:
  PS-Simulink Converter/LConn1 -- Conn1/RConn1

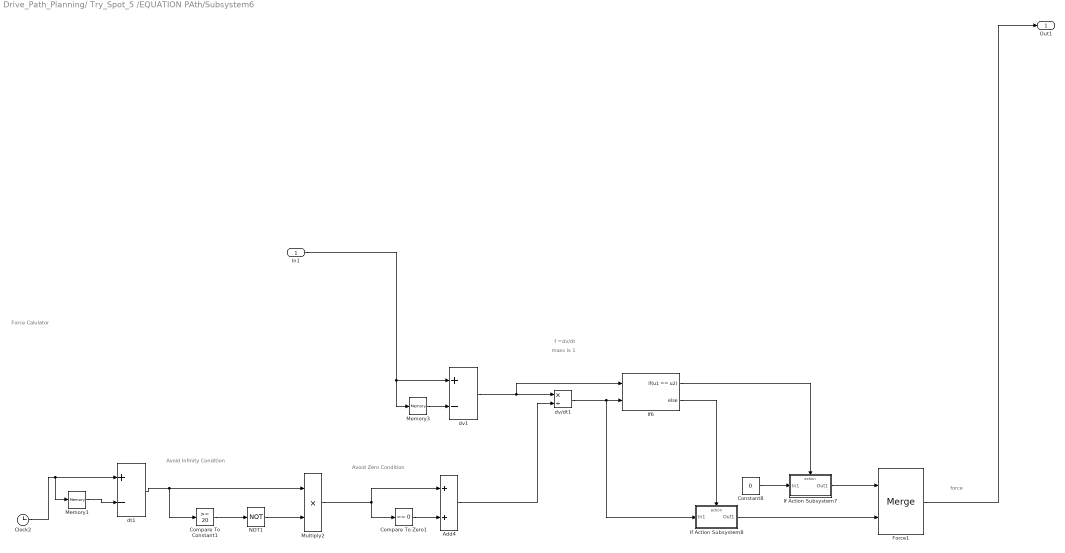
== system Drive_Path_Planning/ Try_Spot_5 /EQUATION PAth/Subsystem6 ==
  note: force
  note: f =dv/dt
  note: Avoid Infinity Condition
  note: Avoid Zero Condition
  note: mass is 1
  note: Force Calulator
  In1 : Inport
  Add4 : Sum
  Clock2 : Clock
  Compare To Constant1 : simulink/Logic and Bit Operations/Compare To Constant  relop=>=  const=20  OutDataTypeStr=boolean
  Compare To Zero1 : simulink/Logic and Bit Operations/Compare To Zero  relop===  OutDataTypeStr=boolean
  Constant8 : Constant  Value=0
  Force1 : Merge
  If Action Subsystem7 : Subsystem  TreatAsAtomicUnit=on
  If Action Subsystem8 : Subsystem  TreatAsAtomicUnit=on
  If6 : If  NumInputs=2  IfExpression=u1 == u2
  Memory1 : Memory
  Memory3 : Memory
  Multiply2 : Product
  NOT1 : Logic  Operator=NOT  IconShape=distinctive  AllPortsSameDT=off  OutDataTypeStr=boolean
  dt1 : Sum  Inputs=+-
  dv/dt1 : Product  Inputs=*/
  dv1 : Sum  Inputs=+-
  Out1 : Outport
  wires:
  Constant8/1 -> If Action Subsystem7/1(In1)
  Compare To Zero1/1 -> Add4/2
  dv1/1 -> If6/1, dv/dt1/1
  Multiply2/1 -> Add4/1, Compare To Zero1/1
  In1/1 -> dv1/1, Memory3/1
  If6/1 -> If Action Subsystem7/Action
  If Action Subsystem8/1(Out1) -> Force1/2
  If6/2 -> If Action Subsystem8/Action
  dv/dt1/1 -> If Action Subsystem8/1(In1), If6/2
  NOT1/1 -> Multiply2/2
  Compare To Constant1/1 -> NOT1/1
  Clock2/1 -> dt1/1, Memory1/1
  Memory1/1 -> dt1/2
  If Action Subsystem7/1(Out1) -> Force1/1
  dt1/1 -> Multiply2/1, Compare To Constant1/1
  Memory3/1 -> dv1/2
  Add4/1 -> dv/dt1/2
  Force1/1 -> Out1/1

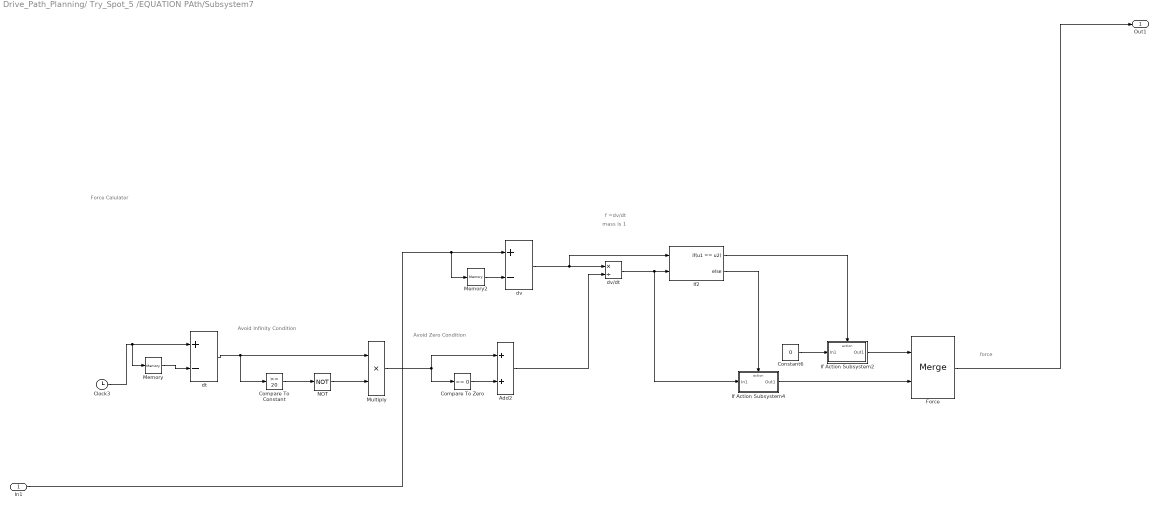
== system Drive_Path_Planning/ Try_Spot_5 /EQUATION PAth/Subsystem7 ==
  note: Force Calulator
  note: f =dv/dt
  note: mass is 1
  note: force
  note: Avoid Infinity Condition
  note: Avoid Zero Condition
  In1 : Inport
  Add2 : Sum
  Clock3 : Clock
  Compare To Constant : simulink/Logic and Bit Operations/Compare To Constant  relop=>=  const=20  OutDataTypeStr=boolean
  Compare To Zero : simulink/Logic and Bit Operations/Compare To Zero  relop===  OutDataTypeStr=boolean
  Constant6 : Constant  Value=0
  Force : Merge
  If Action Subsystem2 : Subsystem  TreatAsAtomicUnit=on
  If Action Subsystem4 : Subsystem  TreatAsAtomicUnit=on
  If2 : If  NumInputs=2  IfExpression=u1 == u2
  Memory : Memory
  Memory2 : Memory
  Multiply : Product
  NOT : Logic  Operator=NOT  IconShape=distinctive  AllPortsSameDT=off  OutDataTypeStr=boolean
  dt : Sum  Inputs=+-
  dv : Sum  Inputs=+-
  dv/dt : Product  Inputs=*/
  Out1 : Outport
  wires:
  If Action Subsystem4/1(Out1) -> Force/2
  dv/dt/1 -> If Action Subsystem4/1(In1), If2/2
  If Action Subsystem2/1(Out1) -> Force/1
  NOT/1 -> Multiply/2
  dt/1 -> Multiply/1, Compare To Constant/1
  Constant6/1 -> If Action Subsystem2/1(In1)
  Multiply/1 -> Add2/1, Compare To Zero/1
  Memory2/1 -> dv/2
  Compare To Zero/1 -> Add2/2
  Compare To Constant/1 -> NOT/1
  Add2/1 -> dv/dt/2
  If2/1 -> If Action Subsystem2/Action
  If2/2 -> If Action Subsystem4/Action
  In1/1 -> Memory2/1, dv/1
  Memory/1 -> dt/2
  dv/1 -> If2/1, dv/dt/1
  Clock3/1 -> dt/1, Memory/1
  Force/1 -> Out1/1

== system Drive_Path_Planning/ Try_Spot_5 /Equation Curve CONSTANT/If Action Subsystem3 ==
  In1 : Inport
  Action Port : ActionPort  ActionPortLabel=if(u1 > 20)
  Out1 : Outport
  wires:
  In1/1 -> Out1/1

== system Drive_Path_Planning/ Try_Spot_5 /Equation Curve CONSTANT/Signal Builder4 ==
  Demux : Demux  Tag=STV Demux  Outputs=1
      settings: DisplayOption=none
  FromWs : FromWorkspace  Tag=STV FromWs  VariableName=tuvar
      SigBuilderData=|
      | common.afterFinalStr = 'Extrapolate'
      | common.sampleTime = 0
      | dataSet.timeRange = [0 30]
      | dataSet.name = 'Group 1'
      | sbobj.Groups.Name = 'Group 1'
      | sbobj.Groups.Signals.Name = 'Signal 1'
      | sbobj.Groups.Signals.XData = [0 20 20 22 22 30]
      | sbobj.Groups.Signals.YData = [0 0 -0.4 -0.4 0 0]
      | sbobj.Groups.TimeRange = [0 30]
  Signal 1 : Outport  Tag=STV Outport
  wires:
  Demux/1 -> Signal 1/1
  FromWs/1 -> Demux/1

== system Drive_Path_Planning/Try_Spot_2 /diagonal return 1/If Action Subsystem ==
  In1 : Inport
  Action Port : ActionPort  ActionPortLabel=if(u1 > 8)
  Out1 : Outport
  wires:
  In1/1 -> Out1/1

== system Drive_Path_Planning/Try_Spot_2 /diagonal return 1/If Action Subsystem1 ==
  In1 : Inport
  Action Port : ActionPort  ActionPortLabel=if(u1 > 8)
  Out1 : Outport
  wires:
  In1/1 -> Out1/1

== system Drive_Path_Planning/Try_Spot_2 /diagonal return 1/Signal Builder1 ==
  Demux : Demux  Tag=STV Demux  Outputs=1
      settings: DisplayOption=none
  FromWs : FromWorkspace  Tag=STV FromWs  VariableName=tuvar
      SigBuilderData=|
      | common.afterFinalStr = 'Extrapolate'
      | common.sampleTime = 0
      | dataSet.timeRange = [0 10]
      | dataSet.name = 'Group 1'
      | sbobj.Groups.Name = 'Group 1'
      | sbobj.Groups.Signals.Name = 'Signal 1'
      | sbobj.Groups.Signals.XData = [0 8 8 9 9 10]
      | sbobj.Groups.Signals.YData = [0 0 -0.63 -0.63 0 0]
  Signal 1 : Outport  Tag=STV Outport
  wires:
  Demux/1 -> Signal 1/1
  FromWs/1 -> Demux/1

== system Drive_Path_Planning/Try_Spot_2 /diagonal return 1/Signal Builder2 ==
  Demux : Demux  Tag=STV Demux  Outputs=1
      settings: DisplayOption=none
  FromWs : FromWorkspace  Tag=STV FromWs  VariableName=tuvar
      SigBuilderData=|
      | common.afterFinalStr = 'Extrapolate'
      | common.sampleTime = 0
      | dataSet.timeRange = [0 10]
      | dataSet.name = 'Group 1'
      | sbobj.Groups.Name = 'Group 1'
      | sbobj.Groups.Signals.Name = 'Signal 1'
      | sbobj.Groups.Signals.XData = [0 8 8 9 9 10]
      | sbobj.Groups.Signals.YData = [0 0 -0.63 -0.63 0 0]
  Signal 1 : Outport  Tag=STV Outport
  wires:
  Demux/1 -> Signal 1/1
  FromWs/1 -> Demux/1

== system Drive_Path_Planning/Try_Spot_2 /diagonal1/If Action Subsystem ==
  In1 : Inport
  Action Port : ActionPort  ActionPortLabel=if(u1 > 5)
  Out1 : Outport
  wires:
  In1/1 -> Out1/1

== system Drive_Path_Planning/Try_Spot_2 /diagonal1/If Action Subsystem1 ==
  In1 : Inport
  Action Port : ActionPort  ActionPortLabel=else
  Out1 : Outport
  wires:
  In1/1 -> Out1/1

== system Drive_Path_Planning/Try_Spot_2 /diagonal1/If Action Subsystem2 ==
  In1 : Inport
  Action Port : ActionPort  ActionPortLabel=if(u1 > 5)
  Out1 : Outport
  wires:
  In1/1 -> Out1/1

== system Drive_Path_Planning/Try_Spot_2 /diagonal1/Signal Builder1 ==
  Demux : Demux  Tag=STV Demux  Outputs=1
      settings: DisplayOption=none
  FromWs : FromWorkspace  Tag=STV FromWs  VariableName=tuvar
      SigBuilderData=|
      | common.afterFinalStr = 'Extrapolate'
      | common.sampleTime = 0
      | dataSet.timeRange = [0 10]
      | dataSet.name = 'Group 1'
      | sbobj.Groups.Name = 'Group 1'
      | sbobj.Groups.Signals.Name = 'Signal 1'
      | sbobj.Groups.Signals.XData = [0 5 5 6 6 10]
      | sbobj.Groups.Signals.YData = [0 0 0.63 0.63 0 0]
  Signal 1 : Outport  Tag=STV Outport
  wires:
  Demux/1 -> Signal 1/1
  FromWs/1 -> Demux/1

== system Drive_Path_Planning/Try_Spot_2 /diagonal1/Signal Builder2 ==
  Demux : Demux  Tag=STV Demux  Outputs=1
      settings: DisplayOption=none
  FromWs : FromWorkspace  Tag=STV FromWs  VariableName=tuvar
      SigBuilderData=|
      | common.afterFinalStr = 'Extrapolate'
      | common.sampleTime = 0
      | dataSet.timeRange = [0 10]
      | dataSet.name = 'Group 1'
      | sbobj.Groups.Name = 'Group 1'
      | sbobj.Groups.Signals.Name = 'Signal 1'
      | sbobj.Groups.Signals.XData = [0 5 5 6 6 10]
      | sbobj.Groups.Signals.YData = [0 -0.005 0.63 0.63 0 0]
  Signal 1 : Outport  Tag=STV Outport
  wires:
  Demux/1 -> Signal 1/1
  FromWs/1 -> Demux/1

== system Drive_Path_Planning/Try_Spot_3 /DIAGONAL 2 Return/If Action Subsystem ==
  In1 : Inport
  Action Port : ActionPort  ActionPortLabel=if(u1 > 16.5)
  Out1 : Outport
  wires:
  In1/1 -> Out1/1

== system Drive_Path_Planning/Try_Spot_3 /DIAGONAL 2 Return/If Action Subsystem1 ==
  In1 : Inport
  Action Port : ActionPort  ActionPortLabel=if(u1 > 16.5)
  Out1 : Outport
  wires:
  In1/1 -> Out1/1

== system Drive_Path_Planning/Try_Spot_3 /DIAGONAL 2 Return/Signal Builder2 ==
  Demux : Demux  Tag=STV Demux  Outputs=1
      settings: DisplayOption=none
  FromWs : FromWorkspace  Tag=STV FromWs  VariableName=tuvar
      SigBuilderData=|
      | common.afterFinalStr = 'Extrapolate'
      | common.sampleTime = 0
      | dataSet.timeRange = [0 20]
      | dataSet.name = 'Group 1'
      | sbobj.Groups.Name = 'Group 1'
      | sbobj.Groups.Signals.Name = 'Signal 1'
      | sbobj.Groups.Signals.XData = [0 16.5 16.5 17.5 17.5 20]
      | sbobj.Groups.Signals.YData = [0 0 -0.53 -0.53 0 0]
      | sbobj.Groups.TimeRange = [0 20]
  Signal 1 : Outport  Tag=STV Outport
  wires:
  FromWs/1 -> Demux/1
  Demux/1 -> Signal 1/1

== system Drive_Path_Planning/Try_Spot_3 /DIAGONAL 2 Return/Signal Builder3 ==
  Demux : Demux  Tag=STV Demux  Outputs=1
      settings: DisplayOption=none
  FromWs : FromWorkspace  Tag=STV FromWs  VariableName=tuvar
      SigBuilderData=|
      | common.afterFinalStr = 'Extrapolate'
      | common.sampleTime = 0
      | dataSet.timeRange = [0 20]
      | dataSet.name = 'Group 1'
      | sbobj.Groups.Name = 'Group 1'
      | sbobj.Groups.Signals.Name = 'Signal 1'
      | sbobj.Groups.Signals.XData = [0 16.5 16.5 17.5 17.5 20]
      | sbobj.Groups.Signals.YData = [0 0 -0.585 -0.585 0 0]
      | sbobj.Groups.TimeRange = [0 20]
  Signal 1 : Outport  Tag=STV Outport
  wires:
  FromWs/1 -> Demux/1
  Demux/1 -> Signal 1/1

== system Drive_Path_Planning/Try_Spot_3 /Diagonal 2/If Action Subsystem ==
  In1 : Inport
  Action Port : ActionPort  ActionPortLabel=if(u1 > 13)
  Out1 : Outport
  wires:
  In1/1 -> Out1/1

== system Drive_Path_Planning/Try_Spot_3 /Diagonal 2/If Action Subsystem1 ==
  In1 : Inport
  Action Port : ActionPort  ActionPortLabel=if(u1 > 13)
  Out1 : Outport
  wires:
  In1/1 -> Out1/1

== system Drive_Path_Planning/Try_Spot_3 /Diagonal 2/Signal Builder1 ==
  Demux : Demux  Tag=STV Demux  Outputs=1
      settings: DisplayOption=none
  FromWs : FromWorkspace  Tag=STV FromWs  VariableName=tuvar
      SigBuilderData=|
      | common.afterFinalStr = 'Extrapolate'
      | common.sampleTime = 0
      | dataSet.timeRange = [0 20]
      | dataSet.name = 'Group 1'
      | sbobj.Groups.Name = 'Group 1'
      | sbobj.Groups.Signals.Name = 'Signal 1'
      | sbobj.Groups.Signals.XData = [0 13 13 14 14 20]
      | sbobj.Groups.Signals.YData = [0 0 0.57 0.57 0 0]
      | sbobj.Groups.TimeRange = [0 20]
  Signal 1 : Outport  Tag=STV Outport
  wires:
  FromWs/1 -> Demux/1
  Demux/1 -> Signal 1/1

== system Drive_Path_Planning/Try_Spot_3 /Diagonal 2/Signal Builder2 ==
  Demux : Demux  Tag=STV Demux  Outputs=1
      settings: DisplayOption=none
  FromWs : FromWorkspace  Tag=STV FromWs  VariableName=tuvar
      SigBuilderData=|
      | common.afterFinalStr = 'Extrapolate'
      | common.sampleTime = 0
      | dataSet.timeRange = [0 20]
      | dataSet.name = 'Group 1'
      | sbobj.Groups.Name = 'Group 1'
      | sbobj.Groups.Signals.Name = 'Signal 1'
      | sbobj.Groups.Signals.XData = [0 13 13 14 14 20]
      | sbobj.Groups.Signals.YData = [0 0 0.6 0.6 0 0]
      | sbobj.Groups.TimeRange = [0 20]
  Signal 1 : Outport  Tag=STV Outport
  wires:
  FromWs/1 -> Demux/1
  Demux/1 -> Signal 1/1

== system Drive_Path_Planning/Try_Spot_4/EQUATION PAth1/If Action Subsystem6 ==
  In1 : Inport
  Action Port : ActionPort  ActionPortLabel=if(u1>20)
  Out1 : Outport
  wires:
  In1/1 -> Out1/1

== system Drive_Path_Planning/Try_Spot_4/EQUATION PAth1/Subsystem5 ==
  Abs : Abs
  Add1 : Sum
  Constant3 : Constant  Value=0.525
  Constant4 : Constant  Value=3.854
  Constant5 : Constant  Value=-2.5
  PS-Simulink Converter : nesl_utility/PS-Simulink Converter  PhysicalDomain=network_engine_domain  SubClassName=ps_output  LeftPortType=input  RightPortType=output  PseudoPeriodic=off  Frequencies=[]  Unit=inherit  AffineConversion=off
  Product3 : Product
  Sqrt : Sqrt  OutputSignalType=real  SaturateOnIntegerOverflow=on
  Subtract : Sum  Inputs=+-
  Conn1 : PMIOPort  Side=Left
  Out1 : Outport
  wires:
  Constant4/1 -> Product3/2
  Sqrt/1 -> Add1/1
  Subtract/1 -> Product3/1
  Product3/1 -> Abs/1
  Abs/1 -> Sqrt/1
  Constant5/1 -> Add1/2
  Constant3/1 -> Subtract/2
  PS-Simulink Converter/1 -> Subtract/1
  Add1/1 -> Out1/1
  connections:
  PS-Simulink Converter/LConn1 -- Conn1/RConn1

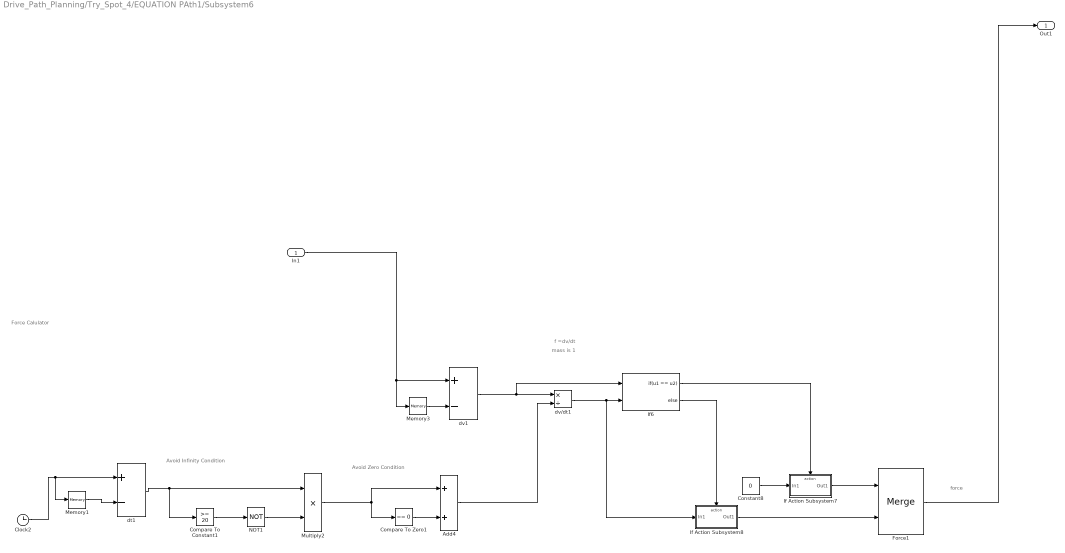
== system Drive_Path_Planning/Try_Spot_4/EQUATION PAth1/Subsystem6 ==
  note: force
  note: f =dv/dt
  note: Avoid Infinity Condition
  note: Avoid Zero Condition
  note: mass is 1
  note: Force Calulator
  In1 : Inport
  Add4 : Sum
  Clock2 : Clock
  Compare To Constant1 : simulink/Logic and Bit Operations/Compare To Constant  relop=>=  const=20  OutDataTypeStr=boolean
  Compare To Zero1 : simulink/Logic and Bit Operations/Compare To Zero  relop===  OutDataTypeStr=boolean
  Constant8 : Constant  Value=0
  Force1 : Merge
  If Action Subsystem7 : Subsystem  TreatAsAtomicUnit=on
  If Action Subsystem8 : Subsystem  TreatAsAtomicUnit=on
  If6 : If  NumInputs=2  IfExpression=u1 == u2
  Memory1 : Memory
  Memory3 : Memory
  Multiply2 : Product
  NOT1 : Logic  Operator=NOT  IconShape=distinctive  AllPortsSameDT=off  OutDataTypeStr=boolean
  dt1 : Sum  Inputs=+-
  dv/dt1 : Product  Inputs=*/
  dv1 : Sum  Inputs=+-
  Out1 : Outport
  wires:
  Constant8/1 -> If Action Subsystem7/1(In1)
  Compare To Zero1/1 -> Add4/2
  dv1/1 -> If6/1, dv/dt1/1
  Multiply2/1 -> Add4/1, Compare To Zero1/1
  In1/1 -> dv1/1, Memory3/1
  If6/1 -> If Action Subsystem7/Action
  If Action Subsystem8/1(Out1) -> Force1/2
  If6/2 -> If Action Subsystem8/Action
  dv/dt1/1 -> If Action Subsystem8/1(In1), If6/2
  NOT1/1 -> Multiply2/2
  Compare To Constant1/1 -> NOT1/1
  Clock2/1 -> dt1/1, Memory1/1
  Memory1/1 -> dt1/2
  If Action Subsystem7/1(Out1) -> Force1/1
  dt1/1 -> Multiply2/1, Compare To Constant1/1
  Memory3/1 -> dv1/2
  Add4/1 -> dv/dt1/2
  Force1/1 -> Out1/1

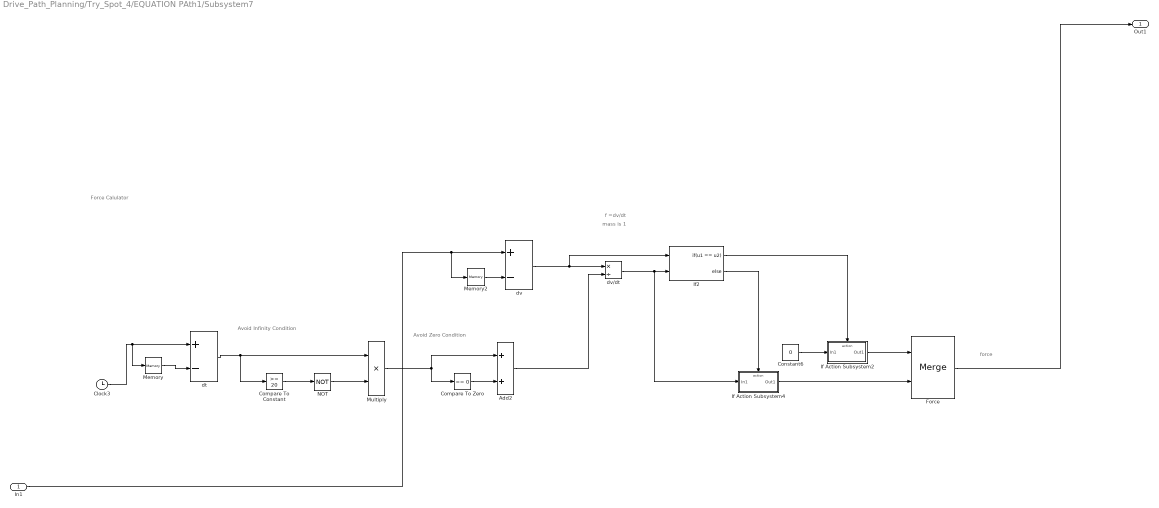
== system Drive_Path_Planning/Try_Spot_4/EQUATION PAth1/Subsystem7 ==
  note: Force Calulator
  note: f =dv/dt
  note: mass is 1
  note: force
  note: Avoid Infinity Condition
  note: Avoid Zero Condition
  In1 : Inport
  Add2 : Sum
  Clock3 : Clock
  Compare To Constant : simulink/Logic and Bit Operations/Compare To Constant  relop=>=  const=20  OutDataTypeStr=boolean
  Compare To Zero : simulink/Logic and Bit Operations/Compare To Zero  relop===  OutDataTypeStr=boolean
  Constant6 : Constant  Value=0
  Force : Merge
  If Action Subsystem2 : Subsystem  TreatAsAtomicUnit=on
  If Action Subsystem4 : Subsystem  TreatAsAtomicUnit=on
  If2 : If  NumInputs=2  IfExpression=u1 == u2
  Memory : Memory
  Memory2 : Memory
  Multiply : Product
  NOT : Logic  Operator=NOT  IconShape=distinctive  AllPortsSameDT=off  OutDataTypeStr=boolean
  dt : Sum  Inputs=+-
  dv : Sum  Inputs=+-
  dv/dt : Product  Inputs=*/
  Out1 : Outport
  wires:
  If Action Subsystem4/1(Out1) -> Force/2
  dv/dt/1 -> If Action Subsystem4/1(In1), If2/2
  If Action Subsystem2/1(Out1) -> Force/1
  NOT/1 -> Multiply/2
  dt/1 -> Multiply/1, Compare To Constant/1
  Constant6/1 -> If Action Subsystem2/1(In1)
  Multiply/1 -> Add2/1, Compare To Zero/1
  Memory2/1 -> dv/2
  Compare To Zero/1 -> Add2/2
  Compare To Constant/1 -> NOT/1
  Add2/1 -> dv/dt/2
  If2/1 -> If Action Subsystem2/Action
  If2/2 -> If Action Subsystem4/Action
  In1/1 -> Memory2/1, dv/1
  Memory/1 -> dt/2
  dv/1 -> If2/1, dv/dt/1
  Clock3/1 -> dt/1, Memory/1
  Force/1 -> Out1/1

== system Drive_Path_Planning/Try_Spot_4/Equation Curve CONSTANT1/If Action Subsystem3 ==
  In1 : Inport
  Action Port : ActionPort  ActionPortLabel=if(u1 > 20)
  Out1 : Outport
  wires:
  In1/1 -> Out1/1

== system Drive_Path_Planning/Try_Spot_4/Equation Curve CONSTANT1/Signal Builder4 ==
  Demux : Demux  Tag=STV Demux  Outputs=1
      settings: DisplayOption=none
  FromWs : FromWorkspace  Tag=STV FromWs  VariableName=tuvar
      SigBuilderData=|
      | common.afterFinalStr = 'Extrapolate'
      | common.sampleTime = 0
      | dataSet.timeRange = [0 30]
      | dataSet.name = 'Group 1'
      | sbobj.Groups.Name = 'Group 1'
      | sbobj.Groups.Signals.Name = 'Signal 1'
      | sbobj.Groups.Signals.XData = [0 20 20 22 22 30]
      | sbobj.Groups.Signals.YData = [0 0 -0.4 -0.4 0 0]
      | sbobj.Groups.TimeRange = [0 30]
  Signal 1 : Outport  Tag=STV Outport
  wires:
  Demux/1 -> Signal 1/1
  FromWs/1 -> Demux/1

== system Drive_Path_Planning/ Try_Spot_5 /EQUATION PAth/Subsystem6/If Action Subsystem7 ==
  In1 : Inport
  Action Port : ActionPort  ActionPortLabel=if(u1 == u2)
  Out1 : Outport  VectorParamsAs1DForOutWhenUnconnected=off
  wires:
  In1/1 -> Out1/1

== system Drive_Path_Planning/ Try_Spot_5 /EQUATION PAth/Subsystem6/If Action Subsystem8 ==
  In1 : Inport
  Action Port : ActionPort  ActionPortLabel=else
  Out1 : Outport  VectorParamsAs1DForOutWhenUnconnected=off
  wires:
  In1/1 -> Out1/1

== system Drive_Path_Planning/ Try_Spot_5 /EQUATION PAth/Subsystem7/If Action Subsystem2 ==
  In1 : Inport
  Action Port : ActionPort  ActionPortLabel=if(u1 == u2)
  Out1 : Outport  VectorParamsAs1DForOutWhenUnconnected=off
  wires:
  In1/1 -> Out1/1

== system Drive_Path_Planning/ Try_Spot_5 /EQUATION PAth/Subsystem7/If Action Subsystem4 ==
  In1 : Inport
  Action Port : ActionPort  ActionPortLabel=else
  Out1 : Outport  VectorParamsAs1DForOutWhenUnconnected=off
  wires:
  In1/1 -> Out1/1

== system Drive_Path_Planning/Try_Spot_4/EQUATION PAth1/Subsystem6/If Action Subsystem7 ==
  In1 : Inport
  Action Port : ActionPort  ActionPortLabel=if(u1 == u2)
  Out1 : Outport  VectorParamsAs1DForOutWhenUnconnected=off
  wires:
  In1/1 -> Out1/1

== system Drive_Path_Planning/Try_Spot_4/EQUATION PAth1/Subsystem6/If Action Subsystem8 ==
  In1 : Inport
  Action Port : ActionPort  ActionPortLabel=else
  Out1 : Outport  VectorParamsAs1DForOutWhenUnconnected=off
  wires:
  In1/1 -> Out1/1

== system Drive_Path_Planning/Try_Spot_4/EQUATION PAth1/Subsystem7/If Action Subsystem2 ==
  In1 : Inport
  Action Port : ActionPort  ActionPortLabel=if(u1 == u2)
  Out1 : Outport  VectorParamsAs1DForOutWhenUnconnected=off
  wires:
  In1/1 -> Out1/1

== system Drive_Path_Planning/Try_Spot_4/EQUATION PAth1/Subsystem7/If Action Subsystem4 ==
  In1 : Inport
  Action Port : ActionPort  ActionPortLabel=else
  Out1 : Outport  VectorParamsAs1DForOutWhenUnconnected=off
  wires:
  In1/1 -> Out1/1
